simulink model "motor_PSD"  (R2024b)
settings: Solver=FixedStepAuto  StartTime=0.0  StopTime=100.0  FixedStep=T_vz  RelTol=1e-3
values from neighbouring files (symbols this model uses):
  Gp_z = c2d(Gp,T_vz)    [main.m]
  q0 = K*(1+(T_vz/(2*Ti))+(Td/T_vz))    [PID_to_PSD.m]    (also in dB_controller.m = u_max)
  q1 = -K*(1+((2*Td)/T_vz)-(T_vz/(2*Ti)))    [PID_to_PSD.m]    (also in dB_controller.m = (a1 - 1)*q0 + 1/b_sum)
  q2 = K*(Td/T_vz)    [PID_to_PSD.m]    (also in dB_controller.m = (a2 - a1)*q0 + a1/b_sum)
  T_vz = 0.01    [main.m]
settings Model: Creator=egoru  LastModifiedBy=tolst

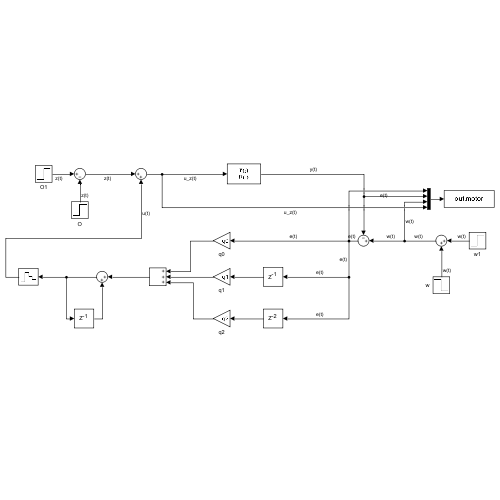
[thumbnail: Simulink's stored preview of the top-level diagram]
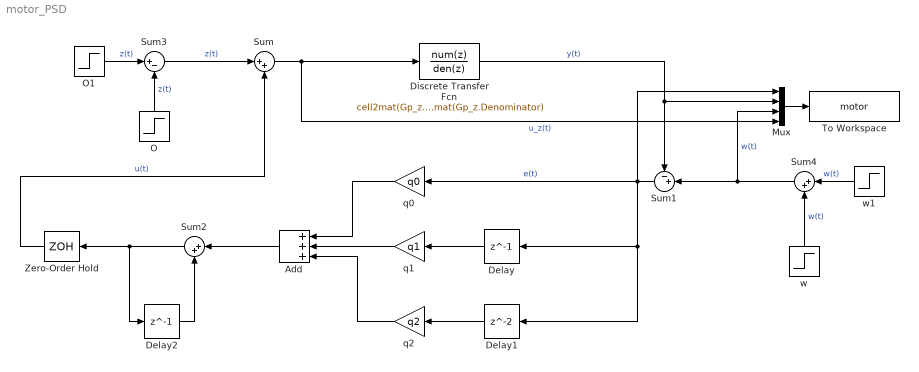
== system motor_PSD ==
  Add : Sum  Inputs=+++
  Delay : Delay  DelayLength=1
  Delay1 : Delay
  Delay2 : Delay  DelayLength=1
  Discrete Transfer Fcn : DiscreteTransferFcn  Numerator=cell2mat(Gp_z.Numerator)  Denominator=cell2mat(Gp_z.Denominator)
  Mux : Mux
  O : Step  Time=50  After=0.2  SampleTime=0
  O1 : Step  Time=40  After=0.2  SampleTime=0
  Sum : Sum  Inputs=|++
  Sum1 : Sum  Inputs=-+|
  Sum2 : Sum  Inputs=|++
  Sum3 : Sum  Inputs=|+-
  Sum4 : Sum  Inputs=|++
  To Workspace : ToWorkspace  VariableName=motor  SaveFormat=Timeseries  SampleTime=-1
  Zero-Order Hold : ZeroOrderHold  SampleTime=T_vz
  q0 : Gain  Gain=q0
  q1 : Gain  Gain=q1
  q2 : Gain  Gain=q2
  w : Step  Time=70  After=-0.2  SampleTime=0
  w1 : Step  Time=10  SampleTime=0
  wires:
  Sum1/1 -> Delay1/1, Delay/1, q0/1, Mux/1  "e(t)"
  Discrete Transfer Fcn/1 -> Mux/2, Sum1/1  "y(t)"
  Mux/1 -> To Workspace/1
  Sum/1 -> Discrete Transfer Fcn/1, Mux/4  "u_z(t)"
  Sum4/1 -> Mux/3, Sum1/2  "w(t)"
  Zero-Order Hold/1 -> Sum/2  "u(t)"
  Delay/1 -> q1/1
  q2/1 -> Add/3
  Sum2/1 -> Zero-Order Hold/1, Delay2/1
  Delay2/1 -> Sum2/2
  Delay1/1 -> q2/1
  q0/1 -> Add/1
  q1/1 -> Add/2
  Add/1 -> Sum2/1
  O1/1 -> Sum3/1  "z(t)"
  Sum3/1 -> Sum/1  "z(t)"
  O/1 -> Sum3/2  "z(t)"
  w/1 -> Sum4/2  "w(t)"
  w1/1 -> Sum4/1  "w(t)"
